simulink model "Power Theft Location"  (R2018a)
settings: Solver=VariableStepAuto  StartTime=0.0  StopTime=1  RelTol=1e-3
libraries: powerlib x20
settings Model: Creator=Sumukh Padalkar  LastModifiedBy=Sumukh Padalkar

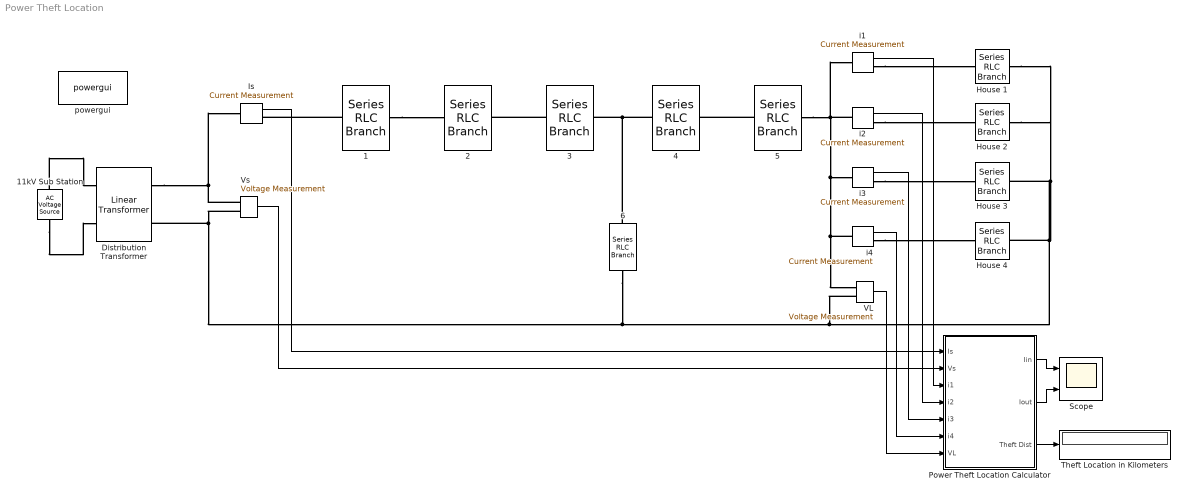
== system Power Theft Location ==
  {1..5} (5 alike) : powerlib/Elements/Series RLC Branch  LConnTagsString=__new0  RConnTagsString=__new0  BranchType=R  Resistance=1  Inductance=0  SetiL0=off  InitialCurrent=0  Capacitance=0  Setx0=off  InitialVoltage=0  Measurements=None  mask(Series RLC Branch){}
      mask Display: image('C:\Users\Sumukh Padalkar\Desktop\unnamed.png');
  11kV Sub Station : powerlib/Electrical Sources/AC Voltage Source  Amplitude=12702.07852  Phase=0  Frequency=50  SampleTime=0  Measurements=None  BusType=swing  Pref=10e3  Qref=0  Qmin=-inf  Qmax=+inf  mask(AC Voltage Source){}
  6 : powerlib/Elements/Series RLC Branch  LConnTagsString=__new0  RConnTagsString=__new0  BranchType=R  Resistance=100  Inductance=0  SetiL0=off  InitialCurrent=0  Capacitance=0  Setx0=off  InitialVoltage=0  Measurements=None
  Distribution Transformer : powerlib/Elements/Linear Transformer  UNITS=SI  NominalPower=[ 17000 50 ]  winding1=[11000 0 0]  winding2=[230 0 0]  ThreeWindings=off  winding3=[3.15e+05 0.7938 0.084225]  RmLm=[inf inf]  Measurements=None  DataType=on
  House 1 : powerlib/Elements/Series RLC Branch  LConnTagsString=__new0  RConnTagsString=__new0  BranchType=R  Resistance=100  Inductance=0  SetiL0=off  InitialCurrent=0  Capacitance=0  Setx0=off  InitialVoltage=0  Measurements=None  mask(Series RLC Branch){}
      mask Display: image('C:\Users\Sumukh Padalkar\Desktop\load.jpg');
  House 2 : powerlib/Elements/Series RLC Branch  LConnTagsString=__new0  RConnTagsString=__new0  BranchType=R  Resistance=100  Inductance=0  SetiL0=off  InitialCurrent=0  Capacitance=0  Setx0=off  InitialVoltage=0  Measurements=None  mask(Series RLC Branch){}
      mask Display: image('C:\Users\Sumukh Padalkar\Desktop\load.jpg');
  House 3 : powerlib/Elements/Series RLC Branch  LConnTagsString=__new0  RConnTagsString=__new0  BranchType=R  Resistance=200  Inductance=0  SetiL0=off  InitialCurrent=0  Capacitance=0  Setx0=off  InitialVoltage=0  Measurements=None  mask(Series RLC Branch){}
      mask Display: image('C:\Users\Sumukh Padalkar\Desktop\load.jpg');
  House 4 : powerlib/Elements/Series RLC Branch  LConnTagsString=__new0  RConnTagsString=__new0  BranchType=R  Resistance=300  Inductance=0  SetiL0=off  InitialCurrent=0  Capacitance=0  Setx0=off  InitialVoltage=0  Measurements=None  mask(Series RLC Branch){}
      mask Display: image('C:\Users\Sumukh Padalkar\Desktop\load.jpg');
  Is : powerlib/Measurements/Current Measurement  PhasorSimulation=off  OutputType=Complex  PSBequivalent=0
  Power Theft Location Calculator : Subsystem
  Scope : Scope  NumInputPorts=2
  Theft Location in Kilometers : Display
      settings: Decimation=15
  VL : powerlib/Measurements/Voltage Measurement  PhasorSimulation=off  OutputType=Complex  PSBequivalent=0
  Vs : powerlib/Measurements/Voltage Measurement  PhasorSimulation=off  OutputType=Complex  PSBequivalent=0
  i{1..4} (4 alike) : powerlib/Measurements/Current Measurement  PhasorSimulation=off  OutputType=Complex  PSBequivalent=0
  powergui : powerlib/powergui  Priority=1  SimulationMode=Continuous  SampleTime=50e-6  frequency=60  Iterations=50  frequencyindice=50  Pbase=100e6  ErrMax=1e-4  UnitsV=kV  UnitsW=MW  buscounter=0  FunctionMessages=off  echomessages=off  EnableUseOfTLC=off  CurrentSourceSwitches=off  DisableSnubberDevices=off  DisableRonSwitches=off  DisableVfSwitches=off  DisplayEquations=off  SolverType=Tustin/Backward Euler (TBE)  Interpol=off  ExternalGateDelay=off  methode=off  Ts=100  x0status=blocks  SPID=on  SwTol=0  HookPort=off  RestoreLinks=warning  ResistiveCurrentMeasurement=off  Frange=[0:2:500]  Ylog=off  Xlog=on  ShowGrid=off  save=off  variable=ZData  structure=0  ZoomFFT=off  StartTime=0.0  cycles=1  DisplayStyle=1  fundamental=60  FreqAxis=off  MaxFrequency=1000  frequencyindicesteady=1  RmsSteady=1  display=off
  wires:
  Power Theft Location Calculator/1(Iin) -> Scope/1
  Power Theft Location Calculator/2(Iout) -> Scope/2
  VL/1 -> Power Theft Location Calculator/7(VL)
  Vs/1 -> Power Theft Location Calculator/2(Vs)
  Is/1 -> Power Theft Location Calculator/1(Is)
  Power Theft Location Calculator/3(Theft Dist) -> Theft Location in Kilometers/1
  i1/1 -> Power Theft Location Calculator/3(i1)
  i2/1 -> Power Theft Location Calculator/4(i2)
  i3/1 -> Power Theft Location Calculator/5(i3)
  i4/1 -> Power Theft Location Calculator/6("i4 ")
  connections:
  11kV Sub Station/RConn1 -- Distribution Transformer/LConn1
  11kV Sub Station/LConn1 -- Distribution Transformer/LConn2
  Distribution Transformer/RConn1 -- Vs/LConn1 -- Is/LConn1
  1/LConn1 -- Is/RConn1
  1/RConn1 -- 2/LConn1
  3/LConn1 -- 2/RConn1
  4/LConn1 -- 3/RConn1 -- 6/LConn1
  i2/RConn1 -- House 2/LConn1
  i3/RConn1 -- House 3/LConn1
  i4/RConn1 -- House 4/LConn1
  i2/LConn1 -- 5/RConn1 -- i1/LConn1 -- i4/LConn1 -- VL/LConn1 -- i3/LConn1
  Vs/LConn2 -- 6/RConn1 -- VL/LConn2 -- House 2/RConn1 -- House 1/RConn1 -- House 3/RConn1 -- House 4/RConn1 -- Distribution Transformer/RConn2
  i1/RConn1 -- House 1/LConn1
  5/LConn1 -- 4/RConn1

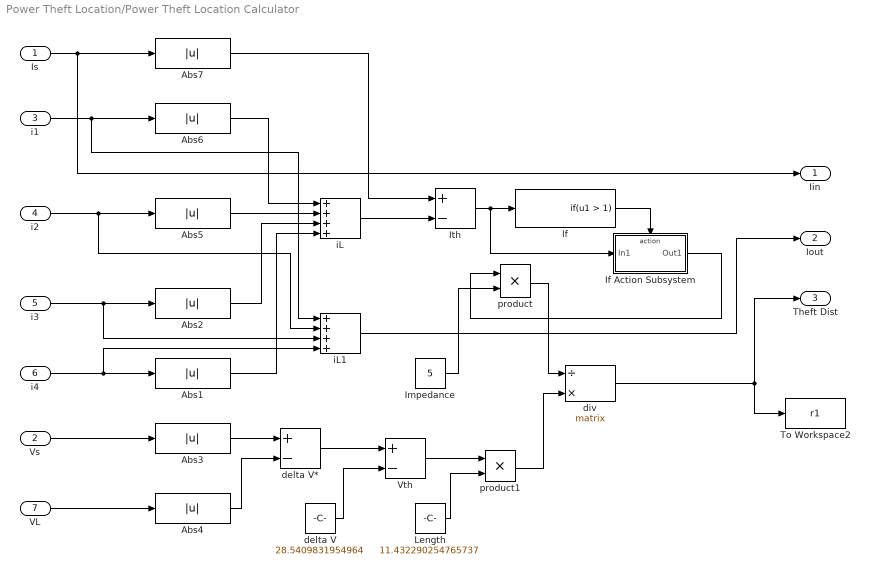
== system Power Theft Location/Power Theft Location Calculator ==
  Is : Inport
  Vs : Inport  Port=2
  i1 : Inport  Port=3
  i2 : Inport  Port=4
  i3 : Inport  Port=5
  "i4 " : Inport  Port=6
  VL : Inport  Port=7
  Abs{1..7} (7 alike) : Abs  ZeroCross=off
  If : If  IfExpression=u1 > 1  ShowElse=off  ZeroCross=off
  If Action Subsystem : Subsystem  TreatAsAtomicUnit=on
  Impedance : Constant  Value=5
  Ith : Sum  Inputs=+-
  Length : Constant  Value=11.432290254765737
  To Workspace2 : ToWorkspace  VariableName=r1  SampleTime=-1
      settings: Save2DSignal=2-D array (concatenate along first dimension)
  Vth : Sum  Inputs=+-
  delta V : Constant  Value=28.5409831954964
  delta V* : Sum  Inputs=+-
  div : Product  Inputs=/*  Multiplication=Matrix(*)
  iL : Sum  Inputs=++++
  iL1 : Sum  Inputs=++++
  "product " : Product
  product1 : Product
  Iin : Outport
  Iout : Outport  Port=2
  Theft Dist : Outport  Port=3
  wires:
  Vth/1 -> product1/1
  Is/1 -> Abs7/1, Iin/1
  Abs1/1 -> iL/4
  iL1/1 -> Iout/1
  "i4 "/1 -> Abs1/1, iL1/4
  delta V/1 -> Vth/2
  Abs5/1 -> iL/2
  VL/1 -> Abs4/1
  Abs7/1 -> Ith/1
  "product "/1 -> div/1
  Abs6/1 -> iL/1
  iL/1 -> Ith/2
  i1/1 -> iL1/1, Abs6/1
  i2/1 -> iL1/2, Abs5/1
  delta V*/1 -> Vth/1
  div/1 -> To Workspace2/1, Theft Dist/1
  Vs/1 -> Abs3/1
  Abs2/1 -> iL/3
  Impedance/1 -> "product "/2
  i3/1 -> Abs2/1, iL1/3
  Abs4/1 -> delta V*/2
  Abs3/1 -> delta V*/1
  Length/1 -> product1/2
  product1/1 -> div/2
  If/1 -> If Action Subsystem/Action
  If Action Subsystem/1(Out1) -> "product "/1
  Ith/1 -> If Action Subsystem/1(In1), If/1

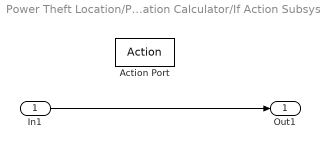
== system Power Theft Location/Power Theft Location Calculator/If Action Subsystem ==
  In1 : Inport
  Action Port : ActionPort  ActionType=then
  Out1 : Outport
  wires:
  In1/1 -> Out1/1
